simulink model "Clase21"  (Simulink 7.2)
settings: Solver=ode45  StartTime=0.0  StopTime=2500  RelTol=1e-3
values from neighbouring files (symbols this model uses):
  A1 = 20    [GlobalParam.m]    (also in GlobalParam2.m = 10)
  A2 = 30    [GlobalParam.m]    (also in GlobalParam2.m = 12)
  R1 = 15    [GlobalParam.m]    (also in GlobalParam2.m)
  R2 = 25    [GlobalParam.m]    (also in GlobalParam2.m = 15)
settings Model: Creator=ALan  LastModifiedBy=ALan

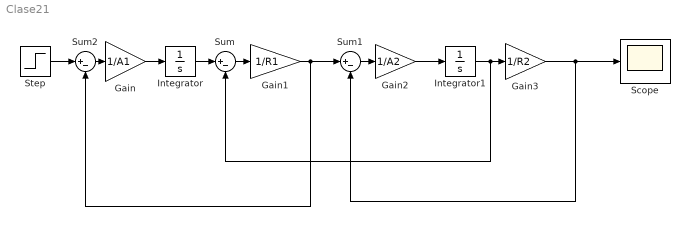
== system Clase21 ==
  Gain : Gain  Gain=1/A1  ParameterDataType=sfix(16)  ParameterScaling=2^0  OutDataType=sfix(16)  OutScaling=2^0
  Gain1 : Gain  Gain=1/R1  ParameterDataType=sfix(16)  ParameterScaling=2^0  OutDataType=sfix(16)  OutScaling=2^0
  Gain2 : Gain  Gain=1/A2  ParameterDataType=sfix(16)  ParameterScaling=2^0  OutDataType=sfix(16)  OutScaling=2^0
  Gain3 : Gain  Gain=1/R2  ParameterDataType=sfix(16)  ParameterScaling=2^0  OutDataType=sfix(16)  OutScaling=2^0
  Integrator : Integrator
  Integrator1 : Integrator
  Scope : Scope
  Step : Step  SampleTime=0
  Sum : Sum  Inputs=|+-  OutDataType=sfix(16)  OutScaling=2^0
  Sum1 : Sum  Inputs=|+-  OutDataType=sfix(16)  OutScaling=2^0
  Sum2 : Sum  Inputs=|+-  OutDataType=sfix(16)  OutScaling=2^0
  wires:
  Sum2/1 -> Gain/1
  Gain/1 -> Integrator/1
  Integrator/1 -> Sum/1
  Sum/1 -> Gain1/1
  Gain1/1 -> Sum1/1, Sum2/2
  Sum1/1 -> Gain2/1
  Gain2/1 -> Integrator1/1
  Integrator1/1 -> Gain3/1, Sum/2
  Gain3/1 -> Sum1/2, Scope/1
  Step/1 -> Sum2/1
